simulink model "UpdateTimeModel"  (R2023b)
settings: Solver=VariableStepAuto  StartTime=0.0  StopTime=10.0  RelTol=1e-3
settings Model: Creator=jsonm  LastModifiedBy=jsonm

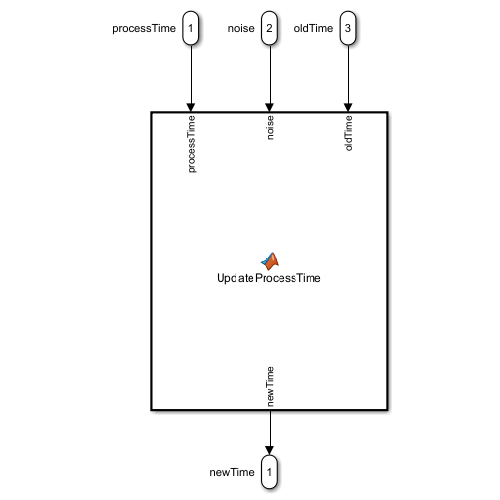
[thumbnail: Simulink's stored preview of the top-level diagram]
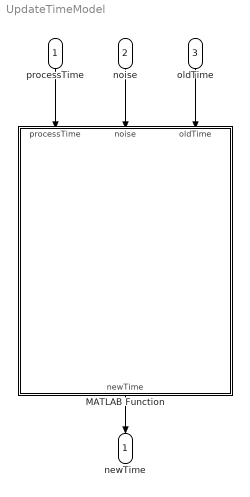
== system UpdateTimeModel ==
  processTime : Inport
  noise : Inport  Port=2
  oldTime : Inport  Port=3
  MATLAB Function : MATLAB Function  TreatAsAtomicUnit=on
  newTime : Outport
  wires:
  processTime/1 -> MATLAB Function/1(processTime)
  noise/1 -> MATLAB Function/2(noise)
  oldTime/1 -> MATLAB Function/3(oldTime)
  MATLAB Function/1(newTime) -> newTime/1

== matlab function UpdateTimeModel/MATLAB Function ==
  data: processTime input; newTime output; noise input; oldTime input
function newTime = UpdateProcessTime(processTime, noise, oldTime)

% Function to update total time based on simple linear model of addition
% assuming CPU times have already been calculated

if nargin < 2
    noise = 0;
    oldTime = 0;
elseif nargin < 3
    oldTime = 0;
end

newTime = oldTime + processTime + noise;
